simulink model "A3_FOPDT_model_set"  (R2023a)
settings: Solver=ode45  StartTime=0.0  StopTime=40  MaxStep=0.5  RelTol=1e-3
values from neighbouring files (symbols this model uses):
  CA0 = 0.9803    [A2_Task9_param_consts.m]
  CAf = 1.0    (= 1)    [A1_find_steady_state.m]    (also in A2_Task9_param_consts.m)
  Cp = 0.239    [A1_find_steady_state.m]    (also in A2_Task9_param_consts.m)
  dHr = -5e4    (= -50000)    [A1_find_steady_state.m]    (also in A2_Task9_param_consts.m)
  ER = 8750    [A1_find_steady_state.m]    (also in A2_Task9_param_consts.m)
  k0 = 6.379829e10    (= 63798290000)    [A1_find_steady_state.m]    (also in A2_Task9_param_consts.m)
  q = 100    [A1_find_steady_state.m]    (also in A2_Task9_param_consts.m)
  rho = 1000    [A1_find_steady_state.m]    (also in A2_Task9_param_consts.m)
  T0 = 303.49    [A2_Task9_param_consts.m]
  Tf = 350    [A1_find_steady_state.m]    (also in A2_Task9_param_consts.m)
  UA = 5e4    (= 50000)    [A1_find_steady_state.m]    (also in A2_Task9_param_consts.m)
  V = 100    [A1_find_steady_state.m]    (also in A2_Task9_param_consts.m)
settings Model: Creator=xiong  LastModifiedBy=xiong

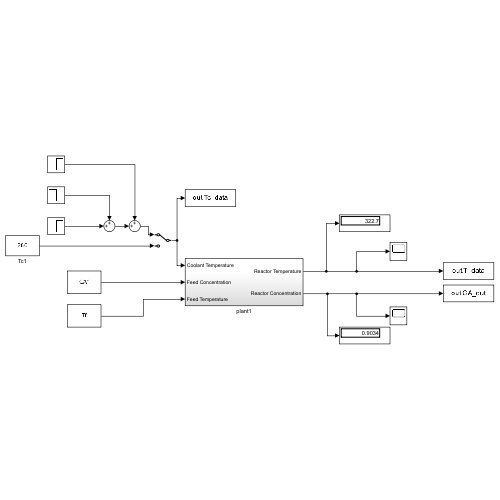
[thumbnail: Simulink's stored preview of the top-level diagram]
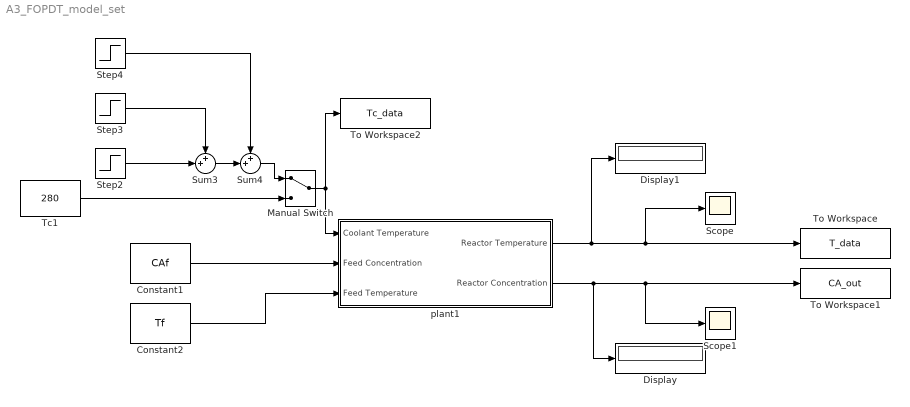
== system A3_FOPDT_model_set ==
  Constant1 : Constant  Value=CAf
  Constant2 : Constant  Value=Tf
  Display : Display
  Display1 : Display
  Manual Switch : ManualSwitch
  Scope : Scope
  Scope1 : Scope
  Step2 : Step  Time=10  Before=280  After=300  SampleTime=0
  Step3 : Step  Time=20  After=-40  SampleTime=0
  Step4 : Step  Time=30  After=40  SampleTime=0
  Sum3 : Sum  Inputs=++|
  Sum4 : Sum  Inputs=++|
  Tc1 : Constant  Value=280
  To Workspace : ToWorkspace  VariableName=T_data  SaveFormat=Structure With Time  SampleTime=-1
  To Workspace1 : ToWorkspace  VariableName=CA_out  SaveFormat=Structure With Time  SampleTime=-1
  To Workspace2 : ToWorkspace  VariableName=Tc_data  SaveFormat=Structure With Time  SampleTime=-1
  plant1 : Subsystem
  wires:
  plant1/1(Reactor Temperature) -> Display1/1, Scope/1, To Workspace/1
  plant1/2(Reactor Concentration) -> Scope1/1, To Workspace1/1, Display/1
  Sum4/1 -> Manual Switch/1
  Constant1/1 -> plant1/2(Feed Concentration)
  Constant2/1 -> plant1/3(Feed Temperature)
  Step2/1 -> Sum3/2
  Step3/1 -> Sum3/1
  Sum3/1 -> Sum4/2
  Step4/1 -> Sum4/1
  Tc1/1 -> Manual Switch/2
  Manual Switch/1 -> plant1/1(Coolant Temperature), To Workspace2/1

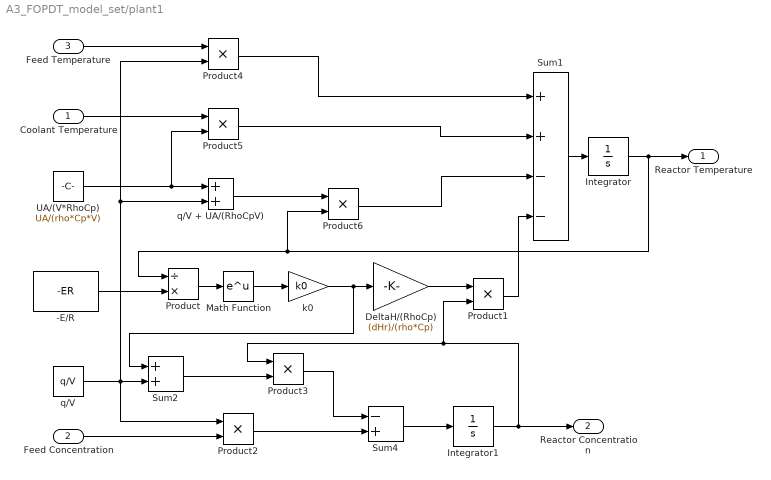
== system A3_FOPDT_model_set/plant1 ==
  Coolant Temperature : Inport
  Feed Concentration : Inport  Port=2
  Feed Temperature : Inport  Port=3
  -E/R : Constant  Value=-ER
  DeltaH/(RhoCp) : Gain  Gain=(dHr)/(rho*Cp)  SaturateOnIntegerOverflow=on  OutDataTypeStr=Inherit: Same as input  ParamDataTypeStr=Inherit: Same as input
  Integrator : Integrator  InitialCondition=T0  LimitOutput=on  LowerSaturationLimit=0
  Integrator1 : Integrator  InitialCondition=CA0  LimitOutput=on  LowerSaturationLimit=0
  Math Function : Math  SignedPower=on
  Product : Product  Inputs=/*  InputSameDT=on  RndMeth=Zero  SaturateOnIntegerOverflow=on  OutDataTypeStr=Inherit: Same as first input
  Product1 : Product  InputSameDT=on  RndMeth=Zero  SaturateOnIntegerOverflow=on  OutDataTypeStr=Inherit: Same as first input
  Product{2,4..6} (4 alike) : Product
  Product3 : Product  InputSameDT=on  RndMeth=Zero  SaturateOnIntegerOverflow=on  OutDataTypeStr=Inherit: Same as first input
  Sum1 : Sum  Inputs=++--  InputSameDT=on  SaturateOnIntegerOverflow=on  OutDataTypeStr=Inherit: Same as first input
  Sum2 : Sum  InputSameDT=on  SaturateOnIntegerOverflow=on  OutDataTypeStr=Inherit: Same as first input
  Sum4 : Sum  Inputs=-+  InputSameDT=on  SaturateOnIntegerOverflow=on  OutDataTypeStr=Inherit: Same as first input
  UA/(V*RhoCp) : Constant  Value=UA/(rho*Cp*V)
  k0 : Gain  Gain=k0  SaturateOnIntegerOverflow=on  OutDataTypeStr=Inherit: Same as input  ParamDataTypeStr=Inherit: Same as input
  q/V : Constant  Value=q/V
  q/V + UA/(RhoCpV) : Sum
  Reactor Temperature : Outport
  Reactor Concentration : Outport  Port=2
  wires:
  Product4/1 -> Sum1/1
  Sum1/1 -> Integrator/1
  Integrator/1 -> Product6/2, Product/1, Reactor Temperature/1
  Product5/1 -> Sum1/2
  Product6/1 -> Sum1/3
  Product/1 -> Math Function/1
  Math Function/1 -> k0/1
  DeltaH/(RhoCp)/1 -> Product1/1
  Product1/1 -> Sum1/4
  k0/1 -> DeltaH/(RhoCp)/1, Sum2/1
  -E/R/1 -> Product/2
  Product3/1 -> Sum4/1
  Sum4/1 -> Integrator1/1
  Integrator1/1 -> Product1/2, Product3/1, Reactor Concentration/1
  q/V/1 -> Product2/1, Sum2/2, Product4/2, q/V + UA/(RhoCpV)/2
  Product2/1 -> Sum4/2
  Feed Temperature/1 -> Product4/1
  Feed Concentration/1 -> Product2/2
  Coolant Temperature/1 -> Product5/1
  Sum2/1 -> Product3/2
  UA/(V*RhoCp)/1 -> Product5/2, q/V + UA/(RhoCpV)/1
  q/V + UA/(RhoCpV)/1 -> Product6/1
